simulink model "second_sim"  (R2020b)
settings: Solver=VariableStepAuto  StartTime=0.0  StopTime=10.0  RelTol=1e-3
undefined symbols (not defined in the file or in its folder): b, k, m
settings Model: Creator=shrin  LastModifiedBy=shrin

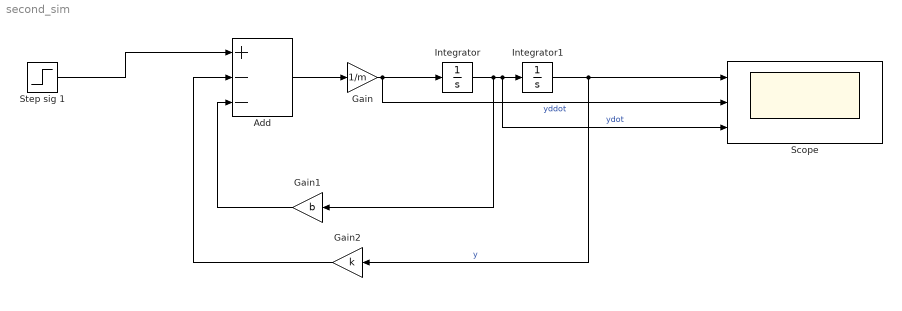
== system second_sim ==
  Add : Sum  Inputs=+--
  Gain : Gain  Gain=1/m
  Gain1 : Gain  Gain=b
  Gain2 : Gain  Gain=k
  Integrator : Integrator  InitialCondition=10
  Integrator1 : Integrator  InitialCondition=20
  Scope : Scope  NumInputPorts=3
  Step sig 1 : Step  Time=5  Before=5  After=10  SampleTime=0
  wires:
  Add/1 -> Gain/1
  Integrator1/1 -> Gain2/1, Scope/1  "y"
  Integrator/1 -> Gain1/1, Scope/3, Integrator1/1  "ydot"
  Gain1/1 -> Add/3
  Gain2/1 -> Add/2
  Step sig 1/1 -> Add/1
  Gain/1 -> Scope/2, Integrator/1  "yddot"
